simulink model "rrm_multibody_cross_validation"  (R2026a)
settings: Solver=ode4  StopTime=rrmStopTime  FixedStep=0.001
model workspace (MAT data in the model file):
  rrmAntiWindupGain = [0.002; 0.002]
  rrmDerivativeAlpha = 0.730402691049
  rrmDqReferenceSignal = timeseries
  rrmDqReferenceSignal.Name = 'unnamed'
  rrmDqReferenceSignal.DataInfo = tsdata.datametadata
  rrmDqReferenceSignal.DataInfo.Interpolation = tsdata.interpolation
  rrmDqReferenceSignal.DataInfo.Interpolation.Fhandle : function handle (value not decoded)
  rrmDqReferenceSignal.DataInfo.Interpolation.Name = 'linear'
  rrmDqReferenceSignal.TimeInfo = tsdata.timemetadata
  rrmDqReferenceSignal.TimeInfo.Length = 31
  rrmDqReferenceSignal.TimeInfo.DuplicateTimes = 0
  rrmDqReferenceSignal.TimeInfo.Time_ = [0; 0.001; 0.002; 0.003; 0.004; 0.005; 0.006; 0.007; 0.008; 0.009; 0.01; 0.011; 0.012; 0.013; 0.014; 0.015; 0.016; 0.017; 0.018; 0.019; 0.02; 0.021; 0.022; 0.023; 0.024; 0.025; 0.026; 0.027; 0.028; 0.029; 0.03]
  rrmDqReferenceSignal.TimeInfo.Initialized = 1
  rrmDqReferenceSignal.QualityInfo = tsdata.qualmetadata
  rrmDqReferenceSignal.Data_ = [0  0; 0.295342434361  0.472547894977; 1.06028752059  1.69646003294; 2.12793814895  3.40470103833; 3.35103216383  5.36165146213; 4.60194236366  7.36310778185; 5.77267650097  9.23628240155; 6.77487728239  10.8398036518; 7.53982236862  12.0637157898; 8.01842437444  12.8294789991; 8.18123086872  13.08996939; 8.01842437444  12.8294789991; 7.53982236862  12.0637157898; 6.77487728239  10.8398036518; 5.77267650097  9.23628240155; 4.60194236366  7.36310778185; 3.35103216383  5.36165146213; 2.12793814895  3.40470103833; 1.06028752059  1.69646003294; 0.295342434361  0.472547894977; 0  0; 0  0; 0  0; 0  0; 0  0; 0  0; 0  0; 0  0; 0  0; 0  0; 0  0]
  rrmInitialDq = [0; 0]
  rrmInitialQ = [0; 0]
  rrmKd = [25; 18]
  rrmKi = [40; 30]
  rrmKp = [120; 100]
  rrmQReferenceSignal = timeseries
  rrmQReferenceSignal.Name = 'unnamed'
  rrmQReferenceSignal.DataInfo = tsdata.datametadata
  rrmQReferenceSignal.DataInfo.Interpolation = tsdata.interpolation
  rrmQReferenceSignal.DataInfo.Interpolation.Fhandle : function handle (value not decoded)
  rrmQReferenceSignal.DataInfo.Interpolation.Name = 'linear'
  rrmQReferenceSignal.TimeInfo = tsdata.timemetadata
  rrmQReferenceSignal.TimeInfo.Length = 31
  rrmQReferenceSignal.TimeInfo.DuplicateTimes = 0
  rrmQReferenceSignal.TimeInfo.Time_ = [0; 0.001; 0.002; 0.003; 0.004; 0.005; 0.006; 0.007; 0.008; 0.009; 0.01; 0.011; 0.012; 0.013; 0.014; 0.015; 0.016; 0.017; 0.018; 0.019; 0.02; 0.021; 0.022; 0.023; 0.024; 0.025; 0.026; 0.027; 0.028; 0.029; 0.03]
  rrmQReferenceSignal.TimeInfo.Initialized = 1
  rrmQReferenceSignal.QualityInfo = tsdata.qualmetadata
  rrmQReferenceSignal.Data_ = [0  0; 0.000101065471998  0.000161704755197; 0.000747000919854  0.00119520147177; 0.0023223241944  0.00371571871103; 0.00505447351378  0.00808715762204; 0.00903344241755  0.0144535078681; 0.0142314147208  0.0227702635532; 0.020522399468  0.0328358391489; 0.0277018658877  0.0443229854202; 0.0355063783456  0.056810205353; 0.0436332312999  0.0698131700798; 0.0517600842541  0.0828161348065; 0.0595645967121  0.0953033547393; 0.0667440631317  0.106790501011; 0.073035047879  0.116856076606; 0.0782330201822  0.125172832291; 0.0822119890859  0.131539182538; 0.0849441384053  0.135910621449; 0.0865194616799  0.138431138688; 0.0871653971277  0.139464635404; 0.0872664625997  0.13962634016; 0.0872664625997  0.13962634016; 0.0872664625997  0.13962634016; 0.0872664625997  0.13962634016; 0.0872664625997  0.13962634016; 0.0872664625997  0.13962634016; 0.0872664625997  0.13962634016; 0.0872664625997  0.13962634016; 0.0872664625997  0.13962634016; 0.0872664625997  0.13962634016; 0.0872664625997  0.13962634016]
  rrmSampleTime = 0.001
  rrmStopTime = 0.03
  rrmTorqueLimits = [25; 15]
undefined symbols (not defined in the file): DiscIntNeverNeededParam
settings Model: Creator=14228  LastModifiedBy=14228

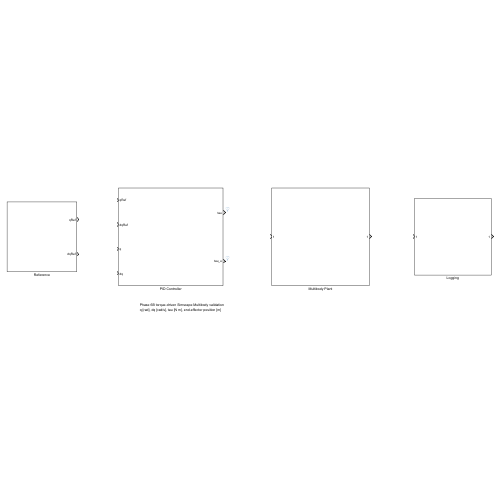
[thumbnail: Simulink's stored preview of the top-level diagram]
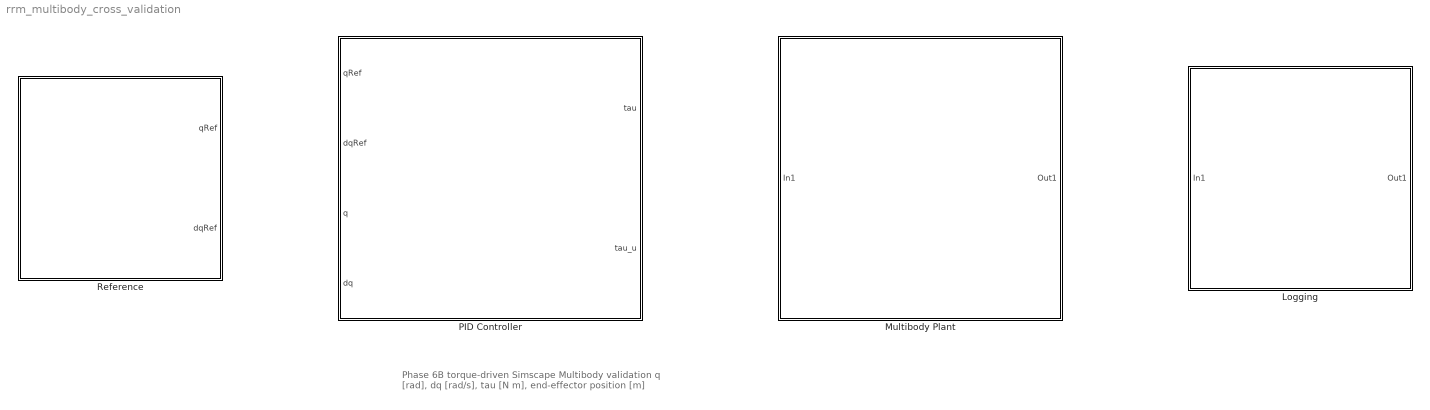
== system rrm_multibody_cross_validation ==
  note: Phase 6B torque-driven Simscape Multibody validation
      | q [rad], dq [rad/s], tau [N m], end-effector position [m]
  Logging : Subsystem
  Multibody Plant : Subsystem
  PID Controller : Subsystem
  Reference : Subsystem

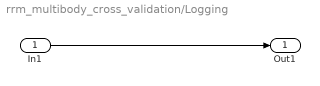
== system rrm_multibody_cross_validation/Logging ==
  In1 : Inport
  Out1 : Outport
  wires:
  In1/1 -> Out1/1

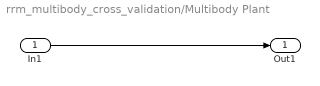
== system rrm_multibody_cross_validation/Multibody Plant ==
  In1 : Inport
  Out1 : Outport
  wires:
  In1/1 -> Out1/1

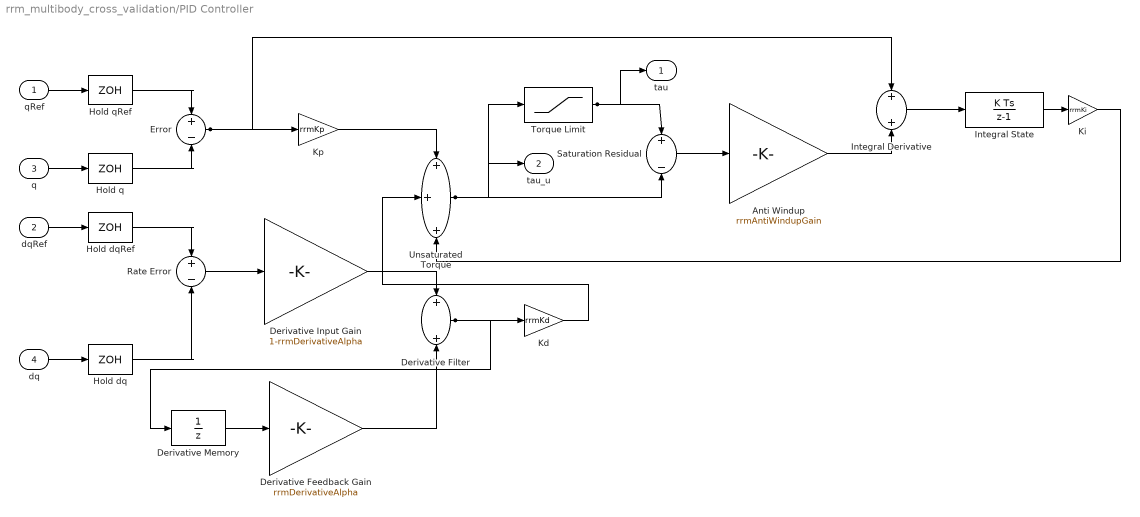
== system rrm_multibody_cross_validation/PID Controller ==
  qRef : Inport
  dqRef : Inport  Port=2
  q : Inport  Port=3
  dq : Inport  Port=4
  Anti Windup : Gain  Gain=rrmAntiWindupGain
  Derivative Feedback Gain : Gain  Gain=rrmDerivativeAlpha
  Derivative Filter : Sum
  Derivative Input Gain : Gain  Gain=1-rrmDerivativeAlpha
  Derivative Memory : UnitDelay  InitialCondition=zeros(2,1)  SampleTime=rrmSampleTime
  Error : Sum  Inputs=+-
  Hold dq : ZeroOrderHold  SampleTime=rrmSampleTime
  Hold dqRef : ZeroOrderHold  SampleTime=rrmSampleTime
  Hold q : ZeroOrderHold  SampleTime=rrmSampleTime
  Hold qRef : ZeroOrderHold  SampleTime=rrmSampleTime
  Integral Derivative : Sum
  Integral State : DiscreteIntegrator  gainval=1  InitialCondition=zeros(2,1)  SampleTime=rrmSampleTime  ICPrevOutput=DiscIntNeverNeededParam  ICPrevScaledInput=DiscIntNeverNeededParam
  Kd : Gain  Gain=rrmKd
  Ki : Gain  Gain=rrmKi
  Kp : Gain  Gain=rrmKp
  Rate Error : Sum  Inputs=+-
  Saturation Residual : Sum  Inputs=+-
  Torque Limit : Saturate  UpperLimit=rrmTorqueLimits  LowerLimit=-rrmTorqueLimits
  Unsaturated Torque : Sum  Inputs=+++
  tau : Outport
  tau_u : Outport  Port=2
  wires:
  Integral State/1 -> Ki/1
  Ki/1 -> Unsaturated Torque/3
  Anti Windup/1 -> Integral Derivative/2
  Integral Derivative/1 -> Integral State/1
  Saturation Residual/1 -> Anti Windup/1
  Kd/1 -> Unsaturated Torque/2
  Torque Limit/1 -> tau/1, Saturation Residual/1
  Unsaturated Torque/1 -> Saturation Residual/2, tau_u/1, Torque Limit/1
  Derivative Feedback Gain/1 -> Derivative Filter/2
  Derivative Filter/1 -> Derivative Memory/1, Kd/1
  Derivative Input Gain/1 -> Derivative Filter/1
  Kp/1 -> Unsaturated Torque/1
  Derivative Memory/1 -> Derivative Feedback Gain/1
  Rate Error/1 -> Derivative Input Gain/1
  Error/1 -> Kp/1, Integral Derivative/1
  Hold dq/1 -> Rate Error/2
  Hold q/1 -> Error/2
  Hold dqRef/1 -> Rate Error/1
  qRef/1 -> Hold qRef/1
  q/1 -> Hold q/1
  dqRef/1 -> Hold dqRef/1
  dq/1 -> Hold dq/1
  Hold qRef/1 -> Error/1

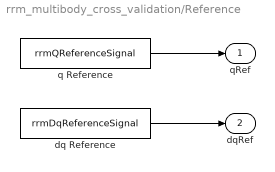
== system rrm_multibody_cross_validation/Reference ==
  dq Reference : FromWorkspace  VariableName=rrmDqReferenceSignal  Interpolate=off  OutputAfterFinalValue=Holding final value
  q Reference : FromWorkspace  VariableName=rrmQReferenceSignal  Interpolate=off  OutputAfterFinalValue=Holding final value
  qRef : Outport
  dqRef : Outport  Port=2
  wires:
  dq Reference/1 -> dqRef/1
  q Reference/1 -> qRef/1
